simulink model "B2_comparison_tool"  (R2021b)
settings: Solver=VariableStepAuto  StartTime=0.0  StopTime=10  RelTol=1e-3
values from neighbouring files (symbols this model uses):
  K_act = 50    [A10_simple_plant.m]    (also in A11_setup_script_pprz.m = 20; A1_setup_script.m = 20)
  K_act_inner = K_act*eye(4)    [A11_setup_script_pprz.m]    (also in A1_setup_script.m)
  K_ec_u = 1.5    [A11_setup_script_pprz.m]    (also in A1_setup_script.m = 5)
  K_ec_v = 1.5    [A11_setup_script_pprz.m]    (also in A1_setup_script.m = 5)
  K_ec_w = 1.5    [A11_setup_script_pprz.m]    (also in A1_setup_script.m = 5)
  K_u_d = 2.5    [A11_setup_script_pprz.m]    (also in A1_setup_script.m = 7)
  K_v_d = 2.5    [A11_setup_script_pprz.m]    (also in A1_setup_script.m = 7)
  K_w_d = 2.5    [A11_setup_script_pprz.m]    (also in A1_setup_script.m = 7)
  max_motor_rate = 30000    [A11_setup_script_pprz.m]    (also in A1_setup_script.m)
  max_omega_motor = 11000    [A11_setup_script_pprz.m]    (also in A1_setup_script.m)
  omega_c_motors = 50    [A11_setup_script_pprz.m]    (also in A1_setup_script.m)
  sampling_time = 1/frequency    (= 0.002)    [A11_setup_script_pprz.m]    (also in A12_sim_multi_run.m; A1_setup_script.m; A6_slow_actuator.m)
undefined symbols (not defined in the file or in its folder): K_ec_d_p, K_ec_d_q, K_ec_d_r, K_ec_dd_p, K_ec_dd_q, K_ec_dd_r, K_ec_p, K_ec_q, K_ec_r, K_p, K_p_d, K_p_dd, K_q, K_q_d, K_q_dd, K_r, K_r_d, K_r_dd
libraries: dspinverses x16, simulink_extras x8, aerolibutil x2, sharedutil x2, aerolibbdyn x2, aerolibatmos2 x2
(part 5 of 5)

== matlab function B2_comparison_tool/System 0 - New/INDI Cascaded w// State Compensation on qdd/STATE COMPENSATION BLOCK/Moment Block form Plant - Plant States/Aerodynamic Forces Calculator ==
  data: xd_body input; Fx_body output; yd_body input; zd_body input; Fy_body output; Fz_body output; L_aero output; M_aero output; N_aero output; rho input; r_plate input; l_plate input; Cl output; Cd output; L output; D output; alpha output; beta output
function [Fx_body, Fy_body, Fz_body, L_aero, M_aero, N_aero, Cl, Cd, L, D, alpha, beta] = aero_forces(xd_body,yd_body,zd_body,rho,r_plate,l_plate)
%% Function to estimate the total aerodynamic force acting on the Quad

% initiate values
Fx_body = 0;
Fy_body = 0;
Fz_body = 0;
L_aero = 0;
M_aero = 0;
N_aero = 0;
Cl = 0;
Cd = 0;
L = 0;
D = 0;
beta = 0;

% Find speed vector in path direction
V_t = sqrt(xd_body^2+yd_body^2+zd_body^2);

% Plate area
S_plate = pi*r_plate^2;

% Protection from alpha singularities
if (abs(zd_body) < 0.02 || abs(xd_body) < 0.02)
    alpha = 0;
else
    alpha = atan2(zd_body, xd_body);

% Find the aerodynamics angles between flight path and body orientation

beta = 0;

% Drag Coefficient
Cd = 0.0033*(90+rad2deg(alpha))+0.7;

% Lift Coefficient
Cl = -0.0228*(90+rad2deg(alpha))+2.01;

% Lateral Coefficients
% Cy = 0;

% Calculate actual forces on the body frame
L = 0.5 * rho * V_t^2 * S_plate * Cl;
D = 0.5 * rho * V_t^2 * S_plate * Cd;
% Y = 0.5 * rho * V_t^2 * S_plate * 0;
% Fx_body = (- D * cos(alpha) * cos(beta) + L * sin(alpha) -Y * cos(alpha) * cos(beta))*sign(xd_body);
% Fy_body = Y * cos(beta) - D * sin(beta);
% Fz_body = - L * cos(alpha) - D * sin(alpha) * cos(beta) - Y * sin(alpha) * sin(beta);

Fx_body = (- D*cos(alpha) + L*sin(alpha))*sign(xd_body);
Fy_body = 0;
Fz_body = (L*cos(alpha) - D*sin(alpha));

% Calculate the moment forces acting on the quad
L_aero = 0;
M_aero = l_plate * (D*cos(alpha)-L*sin(alpha));
N_aero = 0;
end

== matlab function B2_comparison_tool/System 0 - New/INDI Cascaded w// State Compensation on qdd/STATE COMPENSATION BLOCK/Moment Block form Plant - Reference States /Aerodynamic Forces Calculator ==
  data: xd_body input; Fx_body output; yd_body input; zd_body input; Fy_body output; Fz_body output; L_aero output; M_aero output; N_aero output; rho input; r_plate input; l_plate input; Cl output; Cd output; L output; D output; alpha output; beta output
function [Fx_body, Fy_body, Fz_body, L_aero, M_aero, N_aero, Cl, Cd, L, D, alpha, beta] = aero_forces(xd_body,yd_body,zd_body,rho,r_plate,l_plate)
%% Function to estimate the total aerodynamic force acting on the Quad

% initiate values
Fx_body = 0;
Fy_body = 0;
Fz_body = 0;
L_aero = 0;
M_aero = 0;
N_aero = 0;
Cl = 0;
Cd = 0;
L = 0;
D = 0;
beta = 0;

% Find speed vector in path direction
V_t = sqrt(xd_body^2+yd_body^2+zd_body^2);

% Plate area
S_plate = pi*r_plate^2;

% Protection from alpha singularities
if (abs(zd_body) < 0.02 || abs(xd_body) < 0.02)
    alpha = 0;
else
    alpha = atan2(zd_body, xd_body);

% Find the aerodynamics angles between flight path and body orientation

beta = 0;

% Drag Coefficient
Cd = 0.0033*(90+rad2deg(alpha))+0.7;

% Lift Coefficient
Cl = -0.0228*(90+rad2deg(alpha))+2.01;

% Lateral Coefficients
% Cy = 0;

% Calculate actual forces on the body frame
L = 0.5 * rho * V_t^2 * S_plate * Cl;
D = 0.5 * rho * V_t^2 * S_plate * Cd;
% Y = 0.5 * rho * V_t^2 * S_plate * 0;
% Fx_body = (- D * cos(alpha) * cos(beta) + L * sin(alpha) -Y * cos(alpha) * cos(beta))*sign(xd_body);
% Fy_body = Y * cos(beta) - D * sin(beta);
% Fz_body = - L * cos(alpha) - D * sin(alpha) * cos(beta) - Y * sin(alpha) * sin(beta);

Fx_body = (- D*cos(alpha) + L*sin(alpha))*sign(xd_body);
Fy_body = 0;
Fz_body = (L*cos(alpha) - D*sin(alpha));

% Calculate the moment forces acting on the quad
L_aero = 0;
M_aero = l_plate * (D*cos(alpha)-L*sin(alpha));
N_aero = 0;
end

== matlab function B2_comparison_tool/System 0 - New/INDI Cascaded w// State Compensation on qdd/STATE COMPENSATION BLOCK/Straight up formula + derivative ==
  data: r_plate input; qd_x output; l_plate input; Iyy input; rho input; u_b input; v_b input; w_b input; alpha input
function qd_x = fcn(r_plate, l_plate, Iyy, rho, u_b, v_b, w_b, alpha)

S_plate = pi*r_plate^2;
V_t = sqrt(u_b^2+v_b^2+w_b^2);
Cd = 0.0033*(90+rad2deg(alpha))+0.7;
Cl = -0.0228*(90+rad2deg(alpha))+2.01;

qd_x = ((rho*S_plate*l_plate)/(2*Iyy))*(Cd*cos(alpha)-Cl*sin(alpha))*(V_t^2);

end

== matlab function B2_comparison_tool/System 0 - New/INDI w// RSPI/MATLAB Function ==
  data: Ixx input; u_out output; Iyy input; Izz input; K_m input; K_t input; Omega_1 input; Omega_2 input; Omega_3 input; Omega_4 input; Phi input; Psi input; Theta input; b input; l input; m input; dv input; desired_u input; max_omega_motor input; max_motor_rate input; sampling_time input; max_iter input
function u_out = control_allocation_simple(Ixx,Iyy,Izz,K_m,K_t,Omega_1,Omega_2,Omega_3,Omega_4,Phi,Psi,Theta,b,l,m,dv,desired_u,max_omega_motor,max_motor_rate,sampling_time,max_iter)

%% Identify and evaluate effectiveness matrix

B_out = zeros(6,4);

B_out(1,1) = -(2*K_t*Omega_1*(sin(Phi)*sin(Psi) + cos(Phi)*cos(Psi)*sin(Theta)))/m;
B_out(1,2) = -(2*K_t*Omega_2*(sin(Phi)*sin(Psi) + cos(Phi)*cos(Psi)*sin(Theta)))/m;
B_out(1,3) = -(2*K_t*Omega_3*(sin(Phi)*sin(Psi) + cos(Phi)*cos(Psi)*sin(Theta)))/m;
B_out(1,4) = -(2*K_t*Omega_4*(sin(Phi)*sin(Psi) + cos(Phi)*cos(Psi)*sin(Theta)))/m;

B_out(2,1) = (2*K_t*Omega_1*(cos(Psi)*sin(Phi) - cos(Phi)*sin(Psi)*sin(Theta)))/m;
B_out(2,2) = (2*K_t*Omega_2*(cos(Psi)*sin(Phi) - cos(Phi)*sin(Psi)*sin(Theta)))/m;
B_out(2,3) = (2*K_t*Omega_3*(cos(Psi)*sin(Phi) - cos(Phi)*sin(Psi)*sin(Theta)))/m;
B_out(2,4) = (2*K_t*Omega_4*(cos(Psi)*sin(Phi) - cos(Phi)*sin(Psi)*sin(Theta)))/m;

B_out(3,1) = -(2*K_t*Omega_1*cos(Phi)*cos(Theta))/m;
B_out(3,2) = -(2*K_t*Omega_2*cos(Phi)*cos(Theta))/m;
B_out(3,3) = -(2*K_t*Omega_3*cos(Phi)*cos(Theta))/m;
B_out(3,4) = -(2*K_t*Omega_4*cos(Phi)*cos(Theta))/m;

B_out(4,1) = -(2*K_t*Omega_1*b)/Ixx;
B_out(4,2) = (2*K_t*Omega_2*b)/Ixx;
B_out(4,3) = (2*K_t*Omega_3*b)/Ixx;
B_out(4,4) = -(2*K_t*Omega_4*b)/Ixx;

B_out(5,1) = (2*K_t*Omega_1*l)/Iyy;
B_out(5,2) = (2*K_t*Omega_2*l)/Iyy;
B_out(5,3) = -(2*K_t*Omega_3*l)/Iyy;
B_out(5,4) = -(2*K_t*Omega_4*l)/Iyy;

B_out(6,1) = (2*K_m*Omega_1)/Izz;
B_out(6,2) = -(2*K_m*Omega_2)/Izz;
B_out(6,3) = (2*K_m*Omega_3)/Izz;
B_out(6,4) = -(2*K_m*Omega_4)/Izz;

% get current u
actual_u = [Omega_1, Omega_2, Omega_3, Omega_4];

% modify pseudo control to mimimize u
dv = dv + B_out * (actual_u' - desired_u);

%% Apply gains to normalize the effectiveness matrix

gain_motor = max_omega_motor/2;
B_out = B_out * gain_motor;

%% Apply RSPI

% build max e min u array
u_max = [max_omega_motor, max_omega_motor, max_omega_motor, max_omega_motor];
u_min = [0,0,0,0];

% get maximum rate
du_rate_max = zeros(1,length(u_max));
du_rate_max(1:4) = max_motor_rate*sampling_time;
du_rate_min = - du_rate_max;

max_du = zeros(1,length(u_max));
min_du = zeros(1,length(u_max));
%Compute the maximum and minimum control input available for each channel: 
for i=1:length(u_max)
    max_du(i) = min( u_max(i) , actual_u(i) + du_rate_max(i));
    min_du(i) = max( u_min(i) , actual_u(i) + du_rate_min(i));
end

max_du =  u_max;
min_du =  u_min;

max_du_scaled = max_du;
min_du_scaled = min_du;
max_du_scaled = max_du_scaled / gain_motor;
min_du_scaled = min_du_scaled / gain_motor;

max_du_scaled = max_du_scaled';
min_du_scaled = min_du_scaled';

sensibility_pseudo_control = 0.001;

% Multiply the pseudo control with the inversion of the control effectiveness to get the control inputs 
B_inv = pinv(B_out);
du_scaled = B_inv * dv; 

B_new = B_out;

locked_actuator = zeros(1,length(u_max));
Scaling_array = ones(1,length(u_max));
reached_pseudo_control = 0;

%Build the scaling array and check for actuator saturation, if so modify the B matrix: 
for i=1:length(u_max)
    if(du_scaled(i) > 0 && locked_actuator(i) == 0)
        Scaling_array(i) = min( 1 , max_du_scaled(i) / du_scaled(i) );        
    elseif(du_scaled(i) < 0 && locked_actuator(i) == 0 )
        Scaling_array(i) = min( 1 , min_du_scaled(i) / du_scaled(i) );
    end     
end

%If we have saturation reduce the control input and prepare for the next iteration 
if( sum(Scaling_array) < length(Scaling_array) )
    %Determine saturated actuators
    locked_actuator( abs(Scaling_array - min(Scaling_array)) < 0.001 ) = 1;
    %Zeroing the column of the effectiveness matrix related to saturated actuators
    B_new(:, locked_actuator == 1 ) = 0;
    %Scale the control input array: 
    du_scaled_s = du_scaled.*min(Scaling_array);
    %Compute the new maximum achievable pseudo control increment associated to the new control input: 
    du_scaled_tot = du_scaled_s;
    dv_ach = B_out * du_scaled_s;

    %Compute the new objective for the pseudo control of the next iteration 
    new_dv = dv - dv_ach;

    %Check if we satisfy the pseudo control with this actuator configuration: 
    if( sum(abs(new_dv)) < sensibility_pseudo_control ) 
        reached_pseudo_control = 1;
    end  

%If we don't saturate just return the actuator increment and that's it    
else
    du_scaled_tot = du_scaled;
    new_dv = dv;
    du_scaled_s = du_scaled.*min(Scaling_array);
end


%Begin the iterative process if we are saturating one of the actuators
j = 1;
while( sum(Scaling_array) < length(Scaling_array) && j <= max_iter && reached_pseudo_control == 0)
    
    %Compute the new control input with the modified B matrix 
    B_new_inv = pinv(B_new);
    du_scaled = B_new_inv * new_dv; 

    %Build the maximum and minimum delta u available for each channel: 
    max_du_scaled = max_du_scaled - du_scaled_s;
    min_du_scaled = min_du_scaled - du_scaled_s;
    
    Scaling_array = ones(1,length(u_max));
    %Build the scaling array and check for actuator saturation, if so modify the B matrix: 
    for i=1:length(u_max)
        if(du_scaled(i) > 0 && locked_actuator(i) == 0)
            Scaling_array(i) = min( 1 , max_du_scaled(i) / du_scaled(i) );        
        elseif(du_scaled(i) < 0 && locked_actuator(i) == 0 )
            Scaling_array(i) = min( 1 , min_du_scaled(i) / du_scaled(i) );
        end     
    end

    %If we have saturation reduce the control input and prepare for the next iteration 
    if(sum(Scaling_array) < length(Scaling_array))
        %Determine saturated actuators
        locked_actuator( abs( Scaling_array - min(Scaling_array)) < 0.01 ) = 1;
        B_new(:, abs( Scaling_array - min(Scaling_array)) < 0.01 ) = 0;
        %Scale the control input array: 
        du_scaled_s = du_scaled.*min(Scaling_array);
        %Compute the new maximum achievable pseudo control increment associated to the new control input: 
        du_scaled_tot = du_scaled_tot + du_scaled_s;
        dv_ach = B_out * du_scaled_s;   

        %Compute the new objective for the pseudo control of the next iteration 
        new_dv = new_dv - dv_ach;

        %Check if we satisfy the pseudo control with this actuator configuration: 
        if( sum(abs(new_dv)) < sensibility_pseudo_control ) 
            reached_pseudo_control = 1;
        end  

    %If we don't saturate just return the actuator increment and that's it    
    else
        du_scaled_tot = du_scaled_tot + du_scaled;
    end    
   
    %Increase the counter: 
    j = j + 1;
    
end

du = du_scaled_tot;
%Scale back the increment to remove the normalization
du = du * gain_motor;

u_out =  du' + desired_u';

end

== matlab function B2_comparison_tool/System 0 - New/Force and Moment Calculation/Forces due to thrust ==
  data: omega_1 input; omega_2 input; F_t_e output; omega_3 input; omega_4 input; R_bg input; K_t input; F_t_b output
function [F_t_e,F_t_b] = F_t(omega_1, omega_2, omega_3, omega_4, R_bg, K_t)

f_1 = [0 0 -K_t * omega_1^2];
f_2 = [0 0 -K_t * omega_2^2]; 
f_3 = [0 0 -K_t * omega_3^2]; 
f_4 = [0 0 -K_t * omega_4^2];

F_t_e = R_bg * (f_1' + f_2' + f_3' + f_4');
F_t_b = (f_1(:,3) + f_2(:,3) + f_3(:,3) + f_4(:,3));

== matlab function B2_comparison_tool/System 0 - New/Force and Moment Calculation/Forces and Moments due to Aerodynamic Forces/Aerodynamic Forces Calculator ==
  data: xd_body input; Fx_body output; yd_body input; zd_body input; Fy_body output; Fz_body output; L_aero output; M_aero output; N_aero output; rho input; r_plate input; l_plate input; Cl output; Cd output; L output; D output; alpha output; beta output
function [Fx_body, Fy_body, Fz_body, L_aero, M_aero, N_aero, Cl, Cd, L, D, alpha, beta] = aero_forces(xd_body,yd_body,zd_body,rho,r_plate,l_plate)
%% Function to estimate the total aerodynamic force acting on the Quad

% initiate values
Fx_body = 0;
Fy_body = 0;
Fz_body = 0;
L_aero = 0;
M_aero = 0;
N_aero = 0;
Cl = 0;
Cd = 0;
L = 0;
D = 0;
beta = 0;

% Find speed vector in path direction
V_t = sqrt(xd_body^2+yd_body^2+zd_body^2);

% Plate area
S_plate = pi*r_plate^2;

% Protection from alpha singularities
if (abs(zd_body) < 0.02 || abs(xd_body) < 0.02)
    alpha = 0;
else
    alpha = atan2(zd_body, xd_body);

% Find the aerodynamics angles between flight path and body orientation

beta = 0;

% Drag Coefficient
Cd = 0.0033*(90+rad2deg(alpha))+0.7;

% Lift Coefficient
Cl = -0.0228*(90+rad2deg(alpha))+2.01;

% Lateral Coefficients
% Cy = 0;

% Calculate actual forces on the body frame
L = 0.5 * rho * V_t^2 * S_plate * Cl;
D = 0.5 * rho * V_t^2 * S_plate * Cd;
% Y = 0.5 * rho * V_t^2 * S_plate * 0;
% Fx_body = (- D * cos(alpha) * cos(beta) + L * sin(alpha) -Y * cos(alpha) * cos(beta))*sign(xd_body);
% Fy_body = Y * cos(beta) - D * sin(beta);
% Fz_body = - L * cos(alpha) - D * sin(alpha) * cos(beta) - Y * sin(alpha) * sin(beta);

Fx_body = (- D*cos(alpha) + L*sin(alpha))*sign(xd_body);
Fy_body = 0;
Fz_body = (L*cos(alpha) - D*sin(alpha));

% Calculate the moment forces acting on the quad
L_aero = 0;
M_aero = l_plate * (D*cos(alpha)-L*sin(alpha));
N_aero = 0;
end

== matlab function B2_comparison_tool/System 0 - New/Force and Moment Calculation/Moments due to thrust ==
  data: omega_1 input; omega_2 input; M_t output; omega_3 input; omega_4 input; K_t input; K_m input; b input; l input
function M_t = M_t(omega_1, omega_2, omega_3, omega_4, K_t, K_m, b, l)

% forces and torques applied by the propellers in the body frame
t_1 = omega_1^2;
t_2 = omega_2^2;
t_3 = omega_3^2;
t_4 = omega_4^2;
omega_vector = [t_1 t_2 t_3 t_4];

% matrix moments
M_t_matrix = [-b*K_t b*K_t b*K_t -b*K_t;
              l*K_t l*K_t -l*K_t -l*K_t;
              K_m -K_m K_m -K_m];

M_t = M_t_matrix * omega_vector';
